simulink model "DC_motor_simulink"  (R2023b)
settings: Solver=VariableStepAuto  StartTime=0.0  StopTime=50  RelTol=1e-3
values from neighbouring files (symbols this model uses):
  Br = 0    [DC_motor_and_Rod.m]
  Jh = 0.6e-6    (= 6e-07)    [DC_motor_and_Rod.m]    (also in linearized_mechanical_model.m)
  Jm = 4e-6 + 0.6e-6    (= 4.6e-06)    [DC_motor_and_Rod.m]
  k = 0    [DC_motor_and_Rod.m]
  Kc = 0.042    [DC_motor_and_Rod.m]
  L = 1.16e-3    (= 0.00116)    [DC_motor_and_Rod.m]
  Ra = 8.4    [DC_motor_and_Rod.m]
libraries: simulink x1
settings Model: Creator=renzo  LastModifiedBy=renzo

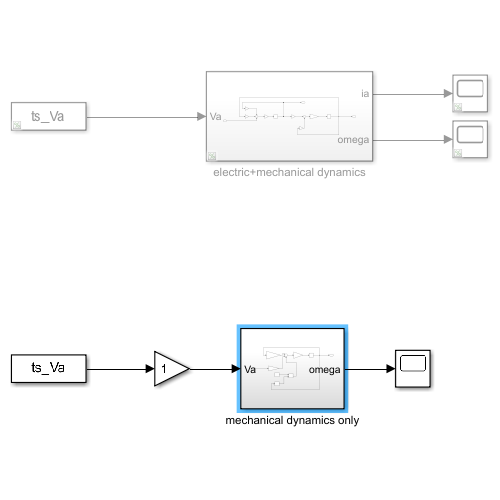
[thumbnail: Simulink's stored preview of the top-level diagram]
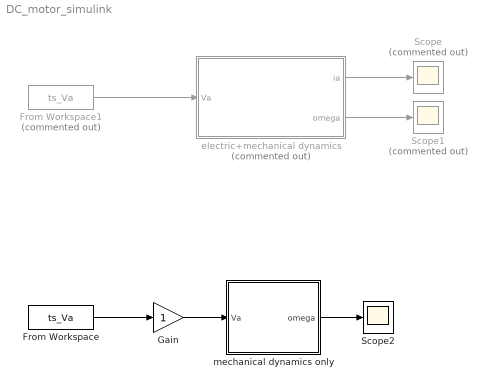
== system DC_motor_simulink ==
  From Workspace : FromWorkspace  VariableName=ts_Va
  From Workspace1 : FromWorkspace  Commented=on  VariableName=ts_Va
  Gain : Gain
  Scope : Scope  Commented=on
  Scope1 : Scope  Commented=on
  Scope2 : Scope
  electric+mechanical dynamics : Subsystem  Commented=on
  mechanical dynamics only : Subsystem
  wires:
  From Workspace1/1 -> electric+mechanical dynamics/1(Va)
  electric+mechanical dynamics/1(ia) -> Scope/1
  electric+mechanical dynamics/2(omega) -> Scope1/1
  From Workspace/1 -> Gain/1
  mechanical dynamics only/1(omega) -> Scope2/1
  Gain/1 -> mechanical dynamics only/1(Va)

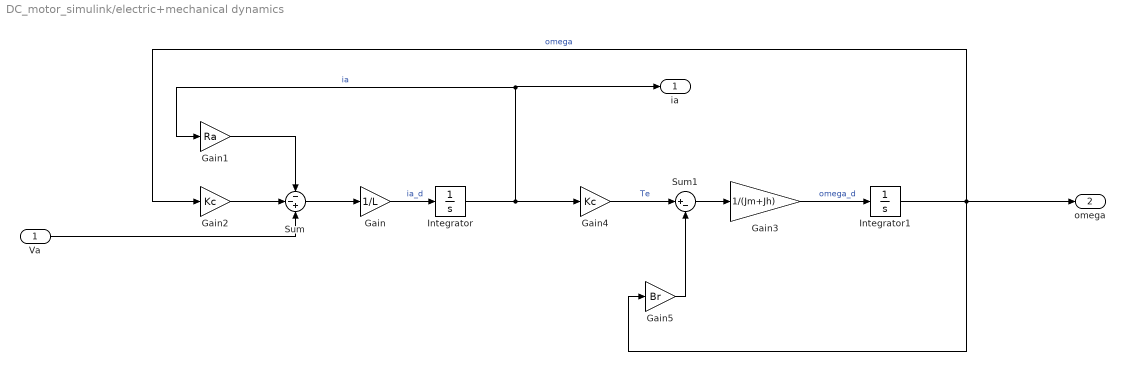
== system DC_motor_simulink/electric+mechanical dynamics ==
  Va : Inport
  Gain : Gain  Gain=1/L
  Gain1 : Gain  Gain=Ra
  Gain2 : Gain  Gain=Kc
  Gain3 : Gain  Gain=1/(Jm+Jh)
  Gain4 : Gain  Gain=Kc
  Gain5 : Gain  Gain=Br
  Integrator : Integrator
  Integrator1 : Integrator
  Sum : Sum  Inputs=--+
  Sum1 : Sum  Inputs=|+-
  ia : Outport
  omega : Outport  Port=2
  wires:
  Gain2/1 -> Sum/2
  Gain1/1 -> Sum/1
  Gain/1 -> Integrator/1  "ia_d"
  Gain4/1 -> Sum1/1  "Te"
  Gain5/1 -> Sum1/2
  Integrator1/1 -> omega/1, Gain2/1, Gain5/1  "omega"
  Integrator/1 -> Gain4/1, ia/1, Gain1/1  "ia"
  Sum/1 -> Gain/1
  Va/1 -> Sum/3
  Sum1/1 -> Gain3/1
  Gain3/1 -> Integrator1/1  "omega_d"

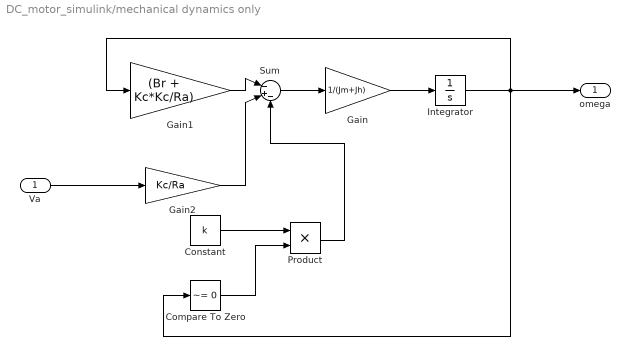
== system DC_motor_simulink/mechanical dynamics only ==
  Va : Inport
  Compare To Zero : simulink/Logic and Bit Operations/Compare To Zero  relop=~=  OutDataTypeStr=boolean
  Constant : Constant  Value=k
  Gain : Gain  Gain=1/(Jm+Jh)
  Gain1 : Gain  Gain=(Br + Kc*Kc/Ra)
  Gain2 : Gain  Gain=Kc/Ra
  Integrator : Integrator
  Product : Product
  Sum : Sum  Inputs=|-+-
  omega : Outport
  wires:
  Sum/1 -> Gain/1
  Gain1/1 -> Sum/1
  Gain2/1 -> Sum/2
  Va/1 -> Gain2/1
  Gain/1 -> Integrator/1
  Constant/1 -> Product/1
  Integrator/1 -> Compare To Zero/1, omega/1, Gain1/1
  Compare To Zero/1 -> Product/2
  Product/1 -> Sum/3
